simulink model "pumaModel"  (R2021b)
settings: Solver=VariableStepAuto  StartTime=0.0  StopTime=stopTime  FixedStep=.0001  RelTol=1e-3
values from neighbouring files (symbols this model uses):
  C = [0 c12_1*dq1 c13_1*dq3;c11_2*dq1 0 c22_2*dq2+c23_2*dq3;c11_3*dq1 c22_3*dq2 0]    [puma560ModifiedDynamics.m]
  dq_0 = [0 0 0]    [matlab.mat]
  fdControl = 2    [InitializationScript.m]
  fEE = 0    [InitializationScript.m]    (also in matlab.mat = 100)
  IC = [0;0;0]    [InitializationScript.m]    (also in matlab.mat = [0 0 0])
  m = 3    [matlab.mat]
  pathPoints = [IC,solution1,solution2,solution3,solution4,solution5,solution6]    [InitializationScript.m]    (also in matlab.mat = [0 0 0 4.71238898038 -1.57079632679 3.14159265359 3.14159265)
  q_0 = [0 0 0]    [matlab.mat]
  timePoints = [0 2 4 6 8 10 12]    [InitializationScript.m]    (also in matlab.mat = [0 2 4 6 8])
  velPoints = zeros(3,7)    [InitializationScript.m]    (also in matlab.mat = [0 0 0 0 0 0 0 0 0 0 0 0 ... (15 elements, 3x5)])
  X = [cos(q1)*(l2*cos(q2)+l3*sin(q2+q3));sin(q1)*(l2*cos(q2)+l3*sin(q2+q3));l1-l2*sin(q2)+l3*cos(q2+q3)]    [puma560ModifiedDynamics.m]
  Y = sym(zeros(3,size(cat(2,Y1,Y2,Y3),2)))    [puma560ModifiedDynamics.m]
undefined symbols (not defined in the file or in its folder): Z
libraries: sm_lib x96, nesl_utility x60, simulink x7, robotmaniplib x1, robotcorelib x1
(part 5 of 5)

== matlab function pumaModel/Controller/Hybrid Motion Force Control/Hybrid Motion Force Control ==
  data: q input; dq input; qd input; dqd input; ddqd input; f input; fd input; Sp input; Sf input; torque output; previousJacOut output; previousJacIn input; test output
function [torque,previousJacOut,test]     = HybridMotionForceControl(q,dq,qd,dqd,ddqd,f,fd,Sp,Sf,previousJacIn)
%% Joint Space variables
q1 = q(1);
q2 = q(2);
q3 = q(3);

dq1 = dq(1);
dq2 = dq(2);
dq3 = dq(3);

qd1 = qd(1);
qd2 = qd(2);
qd3 = qd(3);

%% Manipulator Geometry
l1 = 0.6731;
l2 = 0.432;
l3 = 0.434;
lc2 = 0.216;
lc3 = 0.164;
m2 = 15.46;
m3 = 9.55;
J = 0.302;

J1 = m3 * lc3^2;
J12 = (m2 * lc2^2) + (m3 * l2^2);
J13 = l2 * lc3 * m3;


h11 = J + J1 * (sin(q2 + q3))^2 + J12 * (cos(q2))^2 + 2 * J13 * cos(q2) * sin(q2+q3);
h22 = J1 + J12 + 2 * J13 * sin(q3);
h23 = J1 + J13 * sin(q3);
h32 = h23;
h33 = J1;

H = [h11, 0 ,0 ;
    0 , h22, h23;
    0 , h32, h33];

c12_1 = J1 * sin(2 * (q1 + q2)) - J12 * sin(2 * q2) + 2 * J13 * cos(2 * q2 +q3);
c13_1 = J1 * sin(2 * (q2 + q3)) + 2 * J13 * cos(q2) * cos(q2 + q3);
c11_2 = (1/2) * (-J1 * sin(2 * (q2 + q3)) + J12 * sin(2 * q2) - 2 * J13 * cos(2 * q2 + q3));
c22_2 = 2 * J13 * cos(q3);
c23_2 = J13 * cos(q3);
c22_3 = -J13 * cos(q3)* dq2;%NEED TO CHECK IF THIS IS CORRECT
c11_3 = (-1/2) * (J1 * sin(2 * (q2 + q3)) + J13 * cos(q2) * cos(q2 + q3));

C = [0, c12_1 * dq1, c13_1 * dq3;
    c11_2 * dq1, 0 , (c22_2)* dq2 + (c23_2)*dq3;
    c11_3 * dq1, c22_3 * dq2, 0];

g = 9.81;

g21 = -g * (lc3 * m3 * sin(q2 + q3) + lc2 * m2 * cos(q2) + l2 * m3 * cos(q2));
g31 = -g * (lc3 * m3 * sin(q2 + q3));

G = [0;
    g21;
    g31];

%% Define the Jacobian
jac=[-sin(q1)*(l3*sin(q2 + q3) + l2*cos(q2)), cos(q1)*(l3*cos(q2 + q3) - l2*sin(q2)), l3*cos(q2 + q3)*cos(q1);
 cos(q1)*(l3*sin(q2 + q3) + l2*cos(q2)), sin(q1)*(l3*cos(q2 + q3) - l2*sin(q2)), l3*cos(q2 + q3)*sin(q1);
                                      0,         - l3*sin(q2 + q3) - l2*cos(q2),        -l3*sin(q2 + q3)];
                                  
%% Define the derivative of the jacobian
dJac=[- sin(q1)*(l3*cos(q2 + q3)*(dq2 + dq3) - l2*sin(q2)*dq2) - cos(q1)*(l2*cos(q2) + l3*sin(q2 + q3))*dq1,   sin(q1)*dq1*(l2*sin(q2) - l3*cos(q2 + q3)) - cos(q1)*(l3*sin(q2 + q3)*(dq2 + dq3) + l2*cos(q2)*dq2), - l3*sin(q1)*cos(q2 + q3)*dq1 - l3*cos(q1)*sin(q2 + q3)*(dq2 + dq3);
  cos(q1)*(l3*cos(q2 + q3)*(dq2 + dq3) - l2*sin(q2)*dq2) - sin(q1)*(l2*cos(q2) + l3*sin(q2 + q3))*dq1, - sin(q1)*(l3*sin(q2 + q3)*(dq2 + dq3) + l2*cos(q2)*dq2) - cos(q1)*(l2*sin(q2) - l3*cos(q2 + q3))*dq1,   l3*cos(q1)*cos(q2 + q3)*dq1 - l3*sin(q1)*sin(q2 + q3)*(dq2 + dq3);
                                                                                                                                                                        0,                                                                                    l2*sin(q2)*dq2 - l3*cos(q2 + q3)*(dq2 + dq3),                                                               -l3*cos(q2 + q3)*(dq2 + dq3)];

%% Check to make sure jacobian doesn't hit singularity
%Check to make sure we haven't hit a singularity
if det(jac)<10e-4
    jac=previousJacIn;
    previousJacOut=previousJacIn;
else
    previousJacOut=jac;
end

%% Define the task space matrices
Hp=inv(transpose(jac))*H*inv(jac);
Cp=inv(transpose(jac))*C*inv(jac)-Hp*dJac*inv(jac);
Gp=inv(transpose(jac))*G;

%% Equivalent Task Space Vectors
p=[cos(q1)*(l3*sin(q2 + q3) + l2*cos(q2));sin(q1)*(l3*sin(q2 + q3) + l2*cos(q2));l1 + l3*cos(q2 + q3) - l2*sin(q2)];
pd=[cos(qd1)*(l3*sin(qd2 + qd3) + l2*cos(qd2));sin(qd1)*(l3*sin(qd2 + qd3) + l2*cos(qd2));l1 + l3*cos(qd2 + qd3) - l2*sin(qd2)];

dp=jac*dq;
dpd=jac*dqd;

ddpd=jac*ddqd+dJac*dqd;
                                
%% Function output
%Define the stiffness and damping matrix below for task space directions
Kp=[500 0 0;0 500 0;0 0 500];
Kd=[50 0 0;0 50 0;0 0 50];
Kf=30*eye(3);
R=[0 0 -1;-1 0 0;0 1 0];

Omega_p=R*Sp*transpose(R);
Omega_f=R*Sf*transpose(R);

up=ddpd+Kd*(dpd-dp)+Kp*(pd-p);
uf=fd+Kf*(fd-f)-0*eye(3)*dp;

jacT=transpose(jac);
torque=jacT*(Hp*Omega_p*up+Cp*dp+Gp+Omega_f*uf);

test=[p-pd,f-fd];

== matlab function pumaModel/Controller/HybridImpedanceForceControl/Hybrid Impedance Force Control ==
  data: q input; dq input; ddq input; qd input; dqd input; torque output; ddqd input; f input; fd input
function torque     = ImpedanceControllerTaskSpace_Lectures_NoForceMeasurements(q,dq,ddq,qd,dqd,ddqd,f,fd)
%% Joint Space variables
q1 = q(1);
q2 = q(2);
q3 = q(3);

dq1 = dq(1);
dq2 = dq(2);
dq3 = dq(3);

qd1 = qd(1);
qd2 = qd(2);
qd3 = qd(3);

% dqd1 = dqd(1);
% dqd2 = dqd(2);
% dqd3 = dqd(3);

%% Manipulator Geometry
l1 = 0.6731;
l2 = 0.432;
l3 = 0.434;
lc2 = 0.216;
lc3 = 0.164;
m2 = 15.46;
m3 = 9.55;
J = 0.302;

J1 = m3 * lc3^2;
J12 = (m2 * lc2^2) + (m3 * l2^2);
J13 = l2 * lc3 * m3;


h11 = J + J1 * (sin(q2 + q3))^2 + J12 * (cos(q2))^2 + 2 * J13 * cos(q2) * sin(q2+q3);
h22 = J1 + J12 + 2 * J13 * sin(q3);
h23 = J1 + J13 * sin(q3);
h32 = h23;
h33 = J1;

H = [h11, 0 ,0 ;
    0 , h22, h23;
    0 , h32, h33];

c12_1 = J1 * sin(2 * (q1 + q2)) - J12 * sin(2 * q2) + 2 * J13 * cos(2 * q2 +q3);
c13_1 = J1 * sin(2 * (q2 + q3)) + 2 * J13 * cos(q2) * cos(q2 + q3);
c11_2 = (1/2) * (-J1 * sin(2 * (q2 + q3)) + J12 * sin(2 * q2) - 2 * J13 * cos(2 * q2 + q3));
c22_2 = 2 * J13 * cos(q3);
c23_2 = J13 * cos(q3);
c22_3 = -J13 * cos(q3)* dq2;%NEED TO CHECK IF THIS IS CORRECT
c11_3 = (-1/2) * (J1 * sin(2 * (q2 + q3)) + J13 * cos(q2) * cos(q2 + q3));

C = [0, c12_1 * dq1, c13_1 * dq3;
    c11_2 * dq1, 0 , (c22_2)* dq2 + (c23_2)*dq3;
    c11_3 * dq1, c22_3 * dq2, 0];

g = 9.81;

g21 = -g * (lc3 * m3 * sin(q2 + q3) + lc2 * m2 * cos(q2) + l2 * m3 * cos(q2));
g31 = -g * (lc3 * m3 * sin(q2 + q3));

G = [0;
    g21;
    g31];

%% Define the Jacobian
jac=[-sin(q1)*(l3*sin(q2 + q3) + l2*cos(q2)), cos(q1)*(l3*cos(q2 + q3) - l2*sin(q2)), l3*cos(q2 + q3)*cos(q1);
 cos(q1)*(l3*sin(q2 + q3) + l2*cos(q2)), sin(q1)*(l3*cos(q2 + q3) - l2*sin(q2)), l3*cos(q2 + q3)*sin(q1);
                                      0,         - l3*sin(q2 + q3) - l2*cos(q2),        -l3*sin(q2 + q3)];
                                  
%% Define the derivative of the jacobian
dJac=[- sin(q1)*(l3*cos(q2 + q3)*(dq2 + dq3) - l2*sin(q2)*dq2) - cos(q1)*(l2*cos(q2) + l3*sin(q2 + q3))*dq1,   sin(q1)*dq1*(l2*sin(q2) - l3*cos(q2 + q3)) - cos(q1)*(l3*sin(q2 + q3)*(dq2 + dq3) + l2*cos(q2)*dq2), - l3*sin(q1)*cos(q2 + q3)*dq1 - l3*cos(q1)*sin(q2 + q3)*(dq2 + dq3);
  cos(q1)*(l3*cos(q2 + q3)*(dq2 + dq3) - l2*sin(q2)*dq2) - sin(q1)*(l2*cos(q2) + l3*sin(q2 + q3))*dq1, - sin(q1)*(l3*sin(q2 + q3)*(dq2 + dq3) + l2*cos(q2)*dq2) - cos(q1)*(l2*sin(q2) - l3*cos(q2 + q3))*dq1,   l3*cos(q1)*cos(q2 + q3)*dq1 - l3*sin(q1)*sin(q2 + q3)*(dq2 + dq3);
                                                                                                                                                                        0,                                                                                    l2*sin(q2)*dq2 - l3*cos(q2 + q3)*(dq2 + dq3),                                                               -l3*cos(q2 + q3)*(dq2 + dq3)];

%% Define the task space matrices
Hp=inv(transpose(jac))*H*inv(jac);
Cp=inv(transpose(jac))*C*inv(jac)-Hp*dJac*inv(jac);
Gp=inv(transpose(jac))*G;

%% Equivalent Task Space Vectors
p=[cos(q1)*(l3*sin(q2 + q3) + l2*cos(q2));sin(q1)*(l3*sin(q2 + q3) + l2*cos(q2));l1 + l3*cos(q2 + q3) - l2*sin(q2)];
pd=[cos(qd1)*(l3*sin(qd2 + qd3) + l2*cos(qd2));sin(qd1)*(l3*sin(qd2 + qd3) + l2*cos(qd2));l1 + l3*cos(qd2 + qd3) - l2*sin(qd2)];

dp=jac*dq;
dpd=jac*dqd;

% ddp=jac*ddq+dJac*dq;
ddpd=jac*ddqd+dJac*dqd;
                              
%% Function output
%Define the stiffness and damping matrix below for task space directions
Km=[100 0 0;0 100 0;0 0 100];
Dm=[50 0 0;0 50 0;0 0 50];
Hm=diag([2 2 2]);

jacT=transpose(jac);
u0=inv(Hm)*(-Dm*dp-Km*p+f-fd);
torque=jacT*(Hp*u0+Cp*dp+Gp-f);

== matlab function pumaModel/Controller/HybridImpedanceVelocityControl/Hybrid Impedance Velocity Control ==
  data: q input; dq input; ddq input; qd input; dqd input; torque output; ddqd input; f input
function torque     = ImpedanceVelocityControl(q,dq,ddq,qd,dqd,ddqd,f)
%% Joint Space variables
q1 = q(1);
q2 = q(2);
q3 = q(3);

dq1 = dq(1);
dq2 = dq(2);
dq3 = dq(3);

qd1 = qd(1);
qd2 = qd(2);
qd3 = qd(3);

% dqd1 = dqd(1);
% dqd2 = dqd(2);
% dqd3 = dqd(3);

%% Manipulator Geometry
l1 = 0.6731;
l2 = 0.432;
l3 = 0.434;
lc2 = 0.216;
lc3 = 0.164;
m2 = 15.46;
m3 = 9.55;
J = 0.302;

J1 = m3 * lc3^2;
J12 = (m2 * lc2^2) + (m3 * l2^2);
J13 = l2 * lc3 * m3;


h11 = J + J1 * (sin(q2 + q3))^2 + J12 * (cos(q2))^2 + 2 * J13 * cos(q2) * sin(q2+q3);
h22 = J1 + J12 + 2 * J13 * sin(q3);
h23 = J1 + J13 * sin(q3);
h32 = h23;
h33 = J1;

H = [h11, 0 ,0 ;
    0 , h22, h23;
    0 , h32, h33];

c12_1 = J1 * sin(2 * (q1 + q2)) - J12 * sin(2 * q2) + 2 * J13 * cos(2 * q2 +q3);
c13_1 = J1 * sin(2 * (q2 + q3)) + 2 * J13 * cos(q2) * cos(q2 + q3);
c11_2 = (1/2) * (-J1 * sin(2 * (q2 + q3)) + J12 * sin(2 * q2) - 2 * J13 * cos(2 * q2 + q3));
c22_2 = 2 * J13 * cos(q3);
c23_2 = J13 * cos(q3);
c22_3 = -J13 * cos(q3)* dq2;%NEED TO CHECK IF THIS IS CORRECT
c11_3 = (-1/2) * (J1 * sin(2 * (q2 + q3)) + J13 * cos(q2) * cos(q2 + q3));

C = [0, c12_1 * dq1, c13_1 * dq3;
    c11_2 * dq1, 0 , (c22_2)* dq2 + (c23_2)*dq3;
    c11_3 * dq1, c22_3 * dq2, 0];

g = 9.81;

g21 = -g * (lc3 * m3 * sin(q2 + q3) + lc2 * m2 * cos(q2) + l2 * m3 * cos(q2));
g31 = -g * (lc3 * m3 * sin(q2 + q3));

G = [0;
    g21;
    g31];

%% Define the Jacobian
jac=[-sin(q1)*(l3*sin(q2 + q3) + l2*cos(q2)), cos(q1)*(l3*cos(q2 + q3) - l2*sin(q2)), l3*cos(q2 + q3)*cos(q1);
 cos(q1)*(l3*sin(q2 + q3) + l2*cos(q2)), sin(q1)*(l3*cos(q2 + q3) - l2*sin(q2)), l3*cos(q2 + q3)*sin(q1);
                                      0,         - l3*sin(q2 + q3) - l2*cos(q2),        -l3*sin(q2 + q3)];
                                  
%% Define the derivative of the jacobian
dJac=[- sin(q1)*(l3*cos(q2 + q3)*(dq2 + dq3) - l2*sin(q2)*dq2) - cos(q1)*(l2*cos(q2) + l3*sin(q2 + q3))*dq1,   sin(q1)*dq1*(l2*sin(q2) - l3*cos(q2 + q3)) - cos(q1)*(l3*sin(q2 + q3)*(dq2 + dq3) + l2*cos(q2)*dq2), - l3*sin(q1)*cos(q2 + q3)*dq1 - l3*cos(q1)*sin(q2 + q3)*(dq2 + dq3);
  cos(q1)*(l3*cos(q2 + q3)*(dq2 + dq3) - l2*sin(q2)*dq2) - sin(q1)*(l2*cos(q2) + l3*sin(q2 + q3))*dq1, - sin(q1)*(l3*sin(q2 + q3)*(dq2 + dq3) + l2*cos(q2)*dq2) - cos(q1)*(l2*sin(q2) - l3*cos(q2 + q3))*dq1,   l3*cos(q1)*cos(q2 + q3)*dq1 - l3*sin(q1)*sin(q2 + q3)*(dq2 + dq3);
                                                                                                                                                                        0,                                                                                    l2*sin(q2)*dq2 - l3*cos(q2 + q3)*(dq2 + dq3),                                                               -l3*cos(q2 + q3)*(dq2 + dq3)];

%% Define the task space matrices
Hp=inv(transpose(jac))*H*inv(jac);
Cp=inv(transpose(jac))*C*inv(jac)-Hp*dJac*inv(jac);
Gp=inv(transpose(jac))*G;

%% Equivalent Task Space Vectors
p=[cos(q1)*(l3*sin(q2 + q3) + l2*cos(q2));sin(q1)*(l3*sin(q2 + q3) + l2*cos(q2));l1 + l3*cos(q2 + q3) - l2*sin(q2)];
pd=[cos(qd1)*(l3*sin(qd2 + qd3) + l2*cos(qd2));sin(qd1)*(l3*sin(qd2 + qd3) + l2*cos(qd2));l1 + l3*cos(qd2 + qd3) - l2*sin(qd2)];

dp=jac*dq;
dpd=jac*dqd;

% ddp=jac*ddq+dJac*dq;
ddpd=jac*ddqd+dJac*dqd;
                                 
%% Function output
%Define the stiffness and damping matrix below for task space directions
Km=[700 0 0;0 700 0;0 0 700];
Dm=[50 0 0;0 50 0;0 0 50];
Hm=diag([2 2 2]);

jacT=transpose(jac);
u0=ddpd+inv(Hm)*(Dm*(dpd-dp)+Km*(pd-p)+f);
torque=jacT*(Hp*u0+Cp*dp+Gp-f);

== matlab function pumaModel/Controller/Sliding Robust Control/MATLAB Function ==
  data: u input; y output
function y = fcn(u)

q1=u(1);
q2=u(2);
q3=u(3);




                                                                                                                                                                                                                                                                                                                             y=[(2500000*2^(1/2)*cos(q1 + pi/4)*(217*sin(q2 + q3) + 216*cos(q2)))/(1605355*sin(q2 + q3)^2 + 15647256*cos(q2)^2 + 8457480*sin(q2 + q3)*cos(q2) + 1887500);
                                                                                                                                                                                                                                                                                     (1250000*(82*cos(q2) + 82*cos(q1)*sin(q2) + 82*sin(q1)*sin(q2) - 217*sin(q2 + q3)*sin(q3) + 217*cos(q2 + q3)*cos(q1)*sin(q3) + 217*cos(q2 + q3)*sin(q1)*sin(q3)))/(1107*(1910*sin(q3)^2 - 2683));
- (((211437*sin(q3))/156250 + 17252611/6250000)*((434*cos(q2 + q3)*cos(q1))/5 - (434*sin(q2 + q3))/5 + (434*cos(q2 + q3)*sin(q1))/5))/((44705604969*sin(q3)^2)/97656250000 - 627985016397/976562500000) - (((211437*sin(q3))/312500 + 321071/1250000)*((434*sin(q2 + q3))/5 + (432*cos(q2))/5 - 200*cos(q1)*((217*cos(q2 + q3))/500 - (54*sin(q2))/125) - 200*sin(q1)*((217*cos(q2 + q3))/500 - (54*sin(q2))/125)))/((44705604969*sin(q3)^2)/97656250000 - 627985016397/976562500000)];

== matlab function pumaModel/Controller/Lyaponuv Control/Lyapanov ==
  data: q input; dq input; qd input; dqd input; torque output; ddqd input
function torque   = InverseDynamicComputedTorque(q,dq,qd,dqd,ddqd)
%% Joint Space variables

q1 = q(1);
q2 = q(2);
q3 = q(3);

dq1 = dq(1);
dq2 = dq(2);
dq3 = dq(3);

%% general physical parameters
l1 = 0.6731;
l2 = 0.432;
l3 = 0.434;
lc2 = 0.216;
lc3 = 0.164;
m2 = 15.46;
m3 = 9.55;
J = 0.302;
%% Inertia Matrix Parameters
J1 = m3 * lc3^2;
J12 = (m2 * lc2^2) + (m3 * l2^2);
J13 = l2 * lc3 * m3;


h11 = J + J1 * (sin(q2 + q3))^2 + J12 * (cos(q2))^2 + 2 * J13 * cos(q2) * sin(q2+q3);
h22 = J1 + J12 + 2 * J13 * sin(q3);
h23 = J1 + J13 * sin(q3);
h32 = h23;
h33 = J1;

H = [h11, 0 ,0 ;
    0 , h22, h23;
    0 , h32, h33];

%% Coriolis Matrix Parameters

c12_1 = J1 * sin(2 * (q1 + q2)) - J12 * sin(2 * q2) + 2 * J13 * cos(2 * q2 +q3);
c13_1 = J1 * sin(2 * (q2 + q3)) + 2 * J13 * cos(q2) * cos(q2 + q3);
c11_2 = (1/2) * (-J1 * sin(2 * (q2 + q3)) + J12 * sin(2 * q2) - 2 * J13 * cos(2 * q2 + q3));
c22_2 = 2 * J13 * cos(q3);
c23_2 = J13 * cos(q3);
c22_3 = -J13 * cos(q3)* dq2;%NEED TO CHECK IF THIS IS CORRECT
c11_3 = (-1/2) * (J1 * sin(2 * (q2 + q3)) + J13 * cos(q2) * cos(q2 + q3));

C = [0, c12_1 * dq1, c13_1 * dq3;
    c11_2 * dq1, 0 , (c22_2)* dq2 + (c23_2)*dq3;
    c11_3 * dq1, c22_3 * dq2, 0];

%% Vector of Potential Forces Parameters

g = 9.81;

g21 = -g * (lc3 * m3 * sin(q2 + q3) + lc2 * m2 * cos(q2) + l2 * m3 * cos(q2));
g31 = -g * (lc3 * m3 * sin(q2 + q3));

G = [0;
    g21;
    g31];

%% Function output
Kd=50*eye(3);
lambda=1*eye(3);
qError=q-qd;
dqError=dq-dqd;
torque = H*(ddqd-lambda*dqError)+C*(dqd-lambda*qError)+G-Kd*(dqError+lambda*qError);

== matlab function pumaModel/Controller/PD + Gravity Compensation/PD + Gravity Compensation/MATLAB Function ==
  data: q input; gTorque output
function gTorque  = gravityTorque(q)
q2=q(2);
q3=q(3);
lc3=0.164;
lc2=0.216;
l2=0.432;
m3=9.55;
m2=15.46;
gTorque=[0;lc3*m3*sin(q2+q3)+lc2*m2*cos(q2)+l2*m3*cos(q2);lc3*m3*sin(q2+q3)]*-9.81;

== matlab function pumaModel/Controller/Joint Space Impedance/ImpedanceControllerJointSpace ==
  data: q input; dq input; ddqd input; qd input; dqd input; torque output
function torque   = ImpedanceControllerJointSpace(q,dq,ddqd,qd,dqd)
%%%%%
% 3-DOF Puma-560 Dynamic Model Function
% H(q)* ddq + C(q) * dq + G = tau + tau_e
% q is 3*1 vector of joint variables (radian)
% H(q) is the inertia matrix
% C(q) is the matrix of Coriolis and centrifugal forces
% G(q) is  the vector of potential forces Parameters
% tau is control torque 
% tau_e is the external torque due to the interaction with the environment
%%%%%

%% Joint Space variables

q1 = q(1);
q2 = q(2);
q3 = q(3);

dq1 = dq(1);
dq2 = dq(2);
dq3 = dq(3);

%% general physical parameters

l1 = 0.6731;
l2 = 0.432;
l3 = 0.434;
lc2 = 0.216;
lc3 = 0.164;
m2 = 15.46;
m3 = 9.55;
J = 0.302;

%% Inertia Matrix Parameters

J1 = m3 * lc3^2;
J12 = (m2 * lc2^2) + (m3 * l2^2);
J13 = l2 * lc3 * m3;


h11 = J + J1 * (sin(q2 + q3))^2 + J12 * (cos(q2))^2 + 2 * J13 * cos(q2) * sin(q2+q3);
h22 = J1 + J12 + 2 * J13 * sin(q3);
h23 = J1 + J13 * sin(q3);
h32 = h23;
h33 = J1;

H = [h11, 0 ,0 ;
    0 , h22, h23;
    0 , h32, h33];

%% Coriolis Matrix Parameters

c12_1 = J1 * sin(2 * (q1 + q2)) - J12 * sin(2 * q2) + 2 * J13 * cos(2 * q2 +q3);
c13_1 = J1 * sin(2 * (q2 + q3)) + 2 * J13 * cos(q2) * cos(q2 + q3);
c11_2 = (1/2) * (-J1 * sin(2 * (q2 + q3)) + J12 * sin(2 * q2) - 2 * J13 * cos(2 * q2 + q3));
c22_2 = 2 * J13 * cos(q3);
c23_2 = J13 * cos(q3);
c22_3 = -J13 * cos(q3)* dq2;%NEED TO CHECK IF THIS IS CORRECT
c11_3 = (-1/2) * (J1 * sin(2 * (q2 + q3)) + J13 * cos(q2) * cos(q2 + q3));

C = [0, c12_1 * dq1, c13_1 * dq3;
    c11_2 * dq1, 0 , (c22_2)* dq2 + (c23_2)*dq3;
    c11_3 * dq1, c22_3 * dq2, 0];

%% Vector of Potential Forces Parameters

g = 9.81;

g21 = -g * (lc3 * m3 * sin(q2 + q3) + lc2 * m2 * cos(q2) + l2 * m3 * cos(q2));
g31 = -g * (lc3 * m3 * sin(q2 + q3));

G = [0;
    g21;
    g31];

%% Function output
%Define the stiffness and damping matrix below
K=[1000 0 0;0 2000 0;0 0 1000];
D=[20 0 0;0 0.1 0;0 0 2];
torque = K*(qd-q)+D*(dqd-dq)+C*dq+G+H*ddqd;

== matlab function pumaModel/Controller/InverseTorque/InverseTorque ==
  data: q input; dq input; qd input; dqd input; torque output; ddqd input
function torque  = InverseDynamicComputedTorque(q,dq,qd,dqd,ddqd)
%% Joint Space variables

q1 = q(1);
q2 = q(2);
q3 = q(3);

dq1 = dq(1);
dq2 = dq(2);
dq3 = dq(3);

%% general physical parameters

l1 = 0.6731;
l2 = 0.432;
l3 = 0.434;
lc2 = 0.216;
lc3 = 0.164;
m2 = 15.46;
m3 = 9.55;
J = 0.302;

%% Inertia Matrix Parameters

J1 = m3 * lc3^2;
J12 = (m2 * lc2^2) + (m3 * l2^2);
J13 = l2 * lc3 * m3;


h11 = J + J1 * (sin(q2 + q3))^2 + J12 * (cos(q2))^2 + 2 * J13 * cos(q2) * sin(q2+q3);
h22 = J1 + J12 + 2 * J13 * sin(q3);
h23 = J1 + J13 * sin(q3);
h32 = h23;
h33 = J1;

H = [h11, 0 ,0 ;
    0 , h22, h23;
    0 , h32, h33];

%% Coriolis Matrix Parameters

c12_1 = J1 * sin(2 * (q1 + q2)) - J12 * sin(2 * q2) + 2 * J13 * cos(2 * q2 +q3);
c13_1 = J1 * sin(2 * (q2 + q3)) + 2 * J13 * cos(q2) * cos(q2 + q3);
c11_2 = (1/2) * (-J1 * sin(2 * (q2 + q3)) + J12 * sin(2 * q2) - 2 * J13 * cos(2 * q2 + q3));
c22_2 = 2 * J13 * cos(q3);
c23_2 = J13 * cos(q3);
c22_3 = -J13 * cos(q3) * dq2;
c11_3 = (-1/2) * (J1 * sin(2 * (q2 + q3)) + J13 * cos(q2) * cos(q2 + q3));

C = [0, c12_1 * dq1, c13_1 * dq3;
    c11_2 * dq1, 0 , (c22_2)* dq2 + (c23_2)*dq3;
    c11_3 * dq1, c22_3 * dq2, 0];

%% Vector of Potential Forces Parameters

g = 9.81;

g21 = -g * (lc3 * m3 * sin(q2 + q3) + lc2 * m2 * cos(q2) + l2 * m3 * cos(q2));
g31 = -g * (lc3 * m3 * sin(q2 + q3));

G = [0;
    g21;
    g31];

%% Function output
Kd=20*eye(3);
Kp=diag([50,50,50]);
torque = H*(ddqd-Kd*(dq-dqd)-Kp*(q-qd))+C*dq+G;

== matlab function pumaModel/Controller/Task Space Impedance/ImpedanceControllerTaskSpace ==
  data: q input; dq input; qd input; dqd input; torque output; ddqd input
function torque    = ImpedanceControllerTaskSpace(q,dq,qd,dqd,ddqd)
%% Joint Space variables

q1 = q(1);
q2 = q(2);
q3 = q(3);

dq1 = dq(1);
dq2 = dq(2);
dq3 = dq(3);

qd1 = qd(1);
qd2 = qd(2);
qd3 = qd(3);

%% general physical parameters

l1 = 0.6731;
l2 = 0.432;
l3 = 0.434;
lc2 = 0.216;
lc3 = 0.164;
m2 = 15.46;
m3 = 9.55;
J = 0.302;

%% Inertia Matrix Parameters

J1 = m3 * lc3^2;
J12 = (m2 * lc2^2) + (m3 * l2^2);
J13 = l2 * lc3 * m3;


h11 = J + J1 * (sin(q2 + q3))^2 + J12 * (cos(q2))^2 + 2 * J13 * cos(q2) * sin(q2+q3);
h22 = J1 + J12 + 2 * J13 * sin(q3);
h23 = J1 + J13 * sin(q3);
h32 = h23;
h33 = J1;

H = [h11, 0 ,0 ;
    0 , h22, h23;
    0 , h32, h33];

%% Coriolis Matrix Parameters

c12_1 = J1 * sin(2 * (q1 + q2)) - J12 * sin(2 * q2) + 2 * J13 * cos(2 * q2 +q3);
c13_1 = J1 * sin(2 * (q2 + q3)) + 2 * J13 * cos(q2) * cos(q2 + q3);
c11_2 = (1/2) * (-J1 * sin(2 * (q2 + q3)) + J12 * sin(2 * q2) - 2 * J13 * cos(2 * q2 + q3));
c22_2 = 2 * J13 * cos(q3);
c23_2 = J13 * cos(q3);
c22_3 = -J13 * cos(q3)* dq2;%NEED TO CHECK IF THIS IS CORRECT
c11_3 = (-1/2) * (J1 * sin(2 * (q2 + q3)) + J13 * cos(q2) * cos(q2 + q3));

C = [0, c12_1 * dq1, c13_1 * dq3;
    c11_2 * dq1, 0 , (c22_2)* dq2 + (c23_2)*dq3;
    c11_3 * dq1, c22_3 * dq2, 0];

%% Vector of Potential Forces Parameters

g = 9.81;

g21 = -g * (lc3 * m3 * sin(q2 + q3) + lc2 * m2 * cos(q2) + l2 * m3 * cos(q2));
g31 = -g * (lc3 * m3 * sin(q2 + q3));

G = [0;
    g21;
    g31];

%% Define the Jacobian along with joint->task position
jac=[-sin(q1)*(l3*sin(q2 + q3) + l2*cos(q2)), cos(q1)*(l3*cos(q2 + q3) - l2*sin(q2)), l3*cos(q2 + q3)*cos(q1);
 cos(q1)*(l3*sin(q2 + q3) + l2*cos(q2)), sin(q1)*(l3*cos(q2 + q3) - l2*sin(q2)), l3*cos(q2 + q3)*sin(q1);
                                      0,         - l3*sin(q2 + q3) - l2*cos(q2),        -l3*sin(q2 + q3)];

xCurrent=[cos(q1)*(l3*sin(q2 + q3) + l2*cos(q2));sin(q1)*(l3*sin(q2 + q3) + l2*cos(q2));l1 + l3*cos(q2 + q3) - l2*sin(q2)];
xDesired=[cos(qd1)*(l3*sin(qd2 + qd3) + l2*cos(qd2));sin(qd1)*(l3*sin(qd2 + qd3) + l2*cos(qd2));l1 + l3*cos(qd2 + qd3) - l2*sin(qd2)];

                                  

%% Function output
%Define the stiffness and damping matrix below for task space directions
K=[100 0 0;0 1000 0;0 0 1000];
D=[50 0 0;0 50 0;0 0 50];
%Need to calculate position & velocity error in task space
xError=xDesired-xCurrent;
dxError=jac*dqd-jac*dq;
xVel=jac*dq;
jacT=transpose(jac);
torque=jacT*K*xError+jacT*D*dxError+H*ddqd+C*dq+G;
% torque=G;

== matlab function pumaModel/Controller/Sliding Adaptive Control/AdaptiveLaw ==
  data: q input; dq input; qd input; dqd input; aHatDot output; ddqd input
function aHatDot  = ImpedanceControllerTaskSpace(q,dq,qd,dqd,ddqd)
%Unpackage the incoming reference/measured states

q1 = q(1);
q2 = q(2);
q3 = q(3);

dq1 = dq(1);
dq2 = dq(2);
dq3 = dq(3);

%Define parameters
lambda=1;
P=1000;

%Define all our own variables
qError=q-qd;
dqError=dq-dqd;

dqr=dqd-lambda*eye(3)*qError;
ddqr=ddqd-lambda*eye(3)*dqError;

dqr1=dqr(1);
dqr2=dqr(2);
dqr3=dqr(3);

ddqr1=ddqr(1);
ddqr2=ddqr(2);
ddqr3=ddqr(3);

S=dqError+lambda*eye(3)*qError;

%Define Y
Y=[ddqr1*cos(q2)^2, ddqr1*sin(q2 + q3)*cos(q2), ddqr1*sin(q2 + q3)^2, ddqr1, dq1*dqr2*sin(2*q1 + 2*q2), dq1*dqr2*cos(2*q2 + q3), dq1*dqr2*sin(2*q2), dq1*dqr2, dq3*dqr3*cos(q2 + q3)*cos(q2), dq3*dqr3*sin(2*q2 + 2*q3),             0,     0,             0,     0,                         0,                       0,                  0,                0,                0,       0,            0,             0,     0,     0,                             0,                         0,                  0,            0;
              0,                          0,                    0,     0,                         0,                       0,                  0,        0,                             0,                         0, ddqr2*sin(q3), ddqr2, ddqr3*sin(q3), ddqr3, dq1*dqr1*sin(2*q2 + 2*q3), dq1*dqr1*cos(2*q2 + q3), dq1*dqr1*sin(2*q2), dq2*dqr3*cos(q3), dq3*dqr3*cos(q3), cos(q2), sin(q2 + q3),             0,     0,     0,                             0,                         0,                  0,            0;
              0,                          0,                    0,     0,                         0,                       0,                  0,        0,                             0,                         0,             0,     0,             0,     0,                         0,                       0,                  0,                0,                0,       0,            0, ddqr2*sin(q3), ddqr2, ddqr3, dq1*dqr1*cos(q2 + q3)*cos(q2), dq1*dqr1*sin(2*q2 + 2*q3), dq2^2*dqr2*cos(q3), sin(q2 + q3)];
 

aHatDot=-P*transpose(Y)*S;

== matlab function pumaModel/Controller/Sliding Adaptive Control/Control Law ==
  data: q input; dq input; qd input; dqd input; torque output; ddqd input; aHat input
function torque  = ImpedanceControllerTaskSpace(q,dq,qd,dqd,ddqd,aHat)
%Unpackage the incoming reference/measured states

q1 = q(1);
q2 = q(2);
q3 = q(3);

dq1 = dq(1);
dq2 = dq(2);
dq3 = dq(3);

qd1 = qd(1);
qd2 = qd(2);
qd3 = qd(3);

dqd1 = dqd(1);
dqd2 = dqd(2);
dqd3 = dqd(3);

ddqd1 = ddqd(1);
ddqd2 = ddqd(2);
ddqd3 = ddqd(3);

qError=q-qd;
dqError=dq-dqd;

%Define parameters
lambda=10*eye(3);
K=10;

dqr=dqd-lambda*qError;
ddqr=ddqd-lambda*dqError;

dqr1=dqr(1);
dqr2=dqr(2);
dqr3=dqr(3);

ddqr1=ddqr(1);
ddqr2=ddqr(2);
ddqr3=ddqr(3);

S=dqError+lambda*qError;

%Define Y
Y=[ddqr1*cos(q2)^2, ddqr1*sin(q2 + q3)*cos(q2), ddqr1*sin(q2 + q3)^2, ddqr1, dq1*dqr2*sin(2*q1 + 2*q2), dq1*dqr2*cos(2*q2 + q3), dq1*dqr2*sin(2*q2), dq1*dqr2, dq3*dqr3*cos(q2 + q3)*cos(q2), dq3*dqr3*sin(2*q2 + 2*q3),             0,     0,             0,     0,                         0,                       0,                  0,                0,                0,       0,            0,             0,     0,     0,                             0,                         0,                  0,            0;
              0,                          0,                    0,     0,                         0,                       0,                  0,        0,                             0,                         0, ddqr2*sin(q3), ddqr2, ddqr3*sin(q3), ddqr3, dq1*dqr1*sin(2*q2 + 2*q3), dq1*dqr1*cos(2*q2 + q3), dq1*dqr1*sin(2*q2), dq2*dqr3*cos(q3), dq3*dqr3*cos(q3), cos(q2), sin(q2 + q3),             0,     0,     0,                             0,                         0,                  0,            0;
              0,                          0,                    0,     0,                         0,                       0,                  0,        0,                             0,                         0,             0,     0,             0,     0,                         0,                       0,                  0,                0,                0,       0,            0, ddqr2*sin(q3), ddqr2, ddqr3, dq1*dqr1*cos(q2 + q3)*cos(q2), dq1*dqr1*sin(2*q2 + 2*q3), dq2^2*dqr2*cos(q3), sin(q2 + q3)];
 

torque=Y*aHat-K*eye(3)*S;
